simulink model "model_params"  (Simulink 10.1)
settings: Solver=FixedStepDiscrete  StartTime=0.0  StopTime=10.0  RelTol=1e-3
settings Model: my_user_defined_string_param=Hello world!  my_user_defined_int_param=102030  Creator=max  LastModifiedBy=MaximeBe
settings DataIOCC: SaveFormat=Dataset
settings OptimizationCC: ZeroExternalMemoryAtStartup=off  ZeroInternalMemoryAtStartup=off  LifeSpan=auto
settings DebuggingCC: UnderspecifiedInitializationDetection=Simplified  MergeDetectMultiDrivingBlocksExec=error  SFUnexpectedBacktrackingDiag=error  SFNoUnconditionalDefaultTransitionDiag=error  SFExecutionAtInitializationDiag=warning
settings HardwareCC: ProdBitPerPointer=64  ProdBitPerSizeT=64  ProdBitPerPtrDiffT=64  ProdLargestAtomicFloat=Float  ProdIntDivRoundTo=Zero  ProdEndianess=LittleEndian  ProdWordSize=64  ProdHWDeviceType=Intel->x86-64 (Windows64)
settings ModelReferenceCC: PropagateSignalLabelsOutOfModel=on
settings RTWCC: Description=Generate an RTMaps component embedding the model  SystemTargetFile=rtmaps.tlc  TemplateMakefile=rtmaps_default_tmf  PostCodeGenCommand=rtmaps_post_code_generation(buildInfo)  RetainRTWFile=on  TargetLang=C++
settings STFCustomTargetCC: ModelReferenceCompliant=off  ConcurrentExecutionCompliant=on  CombineOutputUpdateFcns=on  MultiInstanceERTCode=on  CodeInterfacePackaging=C++ class  CPPClassGenCompliant=on  GRTInterface=off  SystemTargetFile=rtmaps.tlc
settings GRTTargetCC: ModelReferenceCompliant=off  ParMdlRefBuildCompliant=off  CompOptLevelCompliant=off  CombineOutputUpdateFcns=on  MatFileLogging=off  MultiInstanceERTCode=on  CodeInterfacePackaging=C++ class  GRTInterface=off  UseToolchainInfoCompliant=off
settings CPPComponent: GenerateDestructor=on  ExternalIOMemberVisibility=private  GenerateExternalIOAccessMethods=Inlined structure-based method  ParameterMemberVisibility=public  InternalMemberVisibility=private  GenerateParameterAccessMethods=None  GenerateInternalMemberAccessMethods=None  UseOperatorNewForModelRefRegistration=off  IncludeModelTypesInModelClass=on
settings ConfigComp: CovMetricSettings=dwe  CovHtmlReporting=off  CovSaveCumulativeToWorkspaceVar=off  CovSaveSingleToWorkspaceVar=off  CovExternalEMLEnable=on

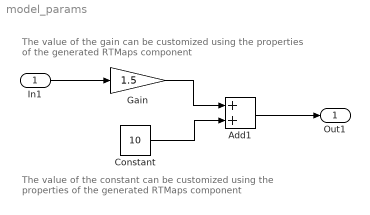
== system model_params ==
  note: The value of the constant can be customized
      | using the properties of the generated RTMaps component
  note: The value of the gain can be customized
      | using the properties of the generated RTMaps component
  In1 : Inport
  Add1 : Sum
  Constant : Constant  Value=10
  Gain : Gain  Gain=1.5
  Out1 : Outport
  wires:
  Add1/1 -> Out1/1
  In1/1 -> Gain/1
  Gain/1 -> Add1/1
  Constant/1 -> Add1/2
